simulink model "EA2_2_regulation_FIXED"  (R2024b)
settings: Solver=VariableStepAuto  StartTime=0.0  StopTime=T_SIM  RelTol=1e-3
values from neighbouring files (symbols this model uses):
  control_par = [k_1, k_2, k_3]    [EA2_2_regulation_FIXED.m]
  controller_index = 2    [EA2_2_regulation_FIXED.m]
  d = d_nominal    (= 0.165)    [EA2_2_regulation_FIXED.m]
  D = diag([0.001, 0.001, 0.0175/6, 0.0175/6, 0.0175/6, 0.0175/6*Ts, 0.0175/6*Ts].^2)    [EA2_2_regulation_FIXED.m]
  d_actual = d_nominal    (= 0.165)    [EA2_2_regulation_FIXED.m]
  ekf_online = 1    [EA2_2_regulation_FIXED.m]
  omega_M = 12    [EA2_2_regulation_FIXED.m]
  P_INIT_EKF = diag([0.001, 0.001, 0.0175/6, 0.0175/6, 0.0175/6, 0.0175/6*Ts, 0.0175/6*Ts].^2)    [EA2_2_regulation_FIXED.m]
  prob_gps_loss = 0    [EA2_2_regulation_FIXED.m]
  q_d = [2;2;0]    [EA2_2_regulation_FIXED.m]
  Q_INIT = [0;0;0]    [EA2_2_regulation_FIXED.m]
  r = r_nominal    (= 0.03)    [EA2_2_regulation_FIXED.m]
  R_2 = diag([ENCODER_QUANTIZATION/6,ENCODER_QUANTIZATION/6].^2)    [EA2_2_regulation_FIXED.m]
  R_5 = diag(([0.001, 0.001, 0.001, ENCODER_QUANTIZATION/6,ENCODER_QUANTIZATION/6]).^2)    [EA2_2_regulation_FIXED.m]
  r_actual = r_nominal    (= 0.03)    [EA2_2_regulation_FIXED.m]
  Ts = 0.04    [EA2_2_regulation_FIXED.m]
  Z_INIT_EKF = [Q_INIT; 0; 0; 0; 0]    [EA2_2_regulation_FIXED.m]
undefined symbols (not defined in the file or in its folder): w_max, X, Y
libraries: robotlib x4
settings Model: Creator=riccardo01  LastModifiedBy=Enrico
settings DataIOCC: SaveFormat=Array  ReturnWorkspaceOutputs=off
settings DebuggingCC: AlgebraicLoopMsg=none

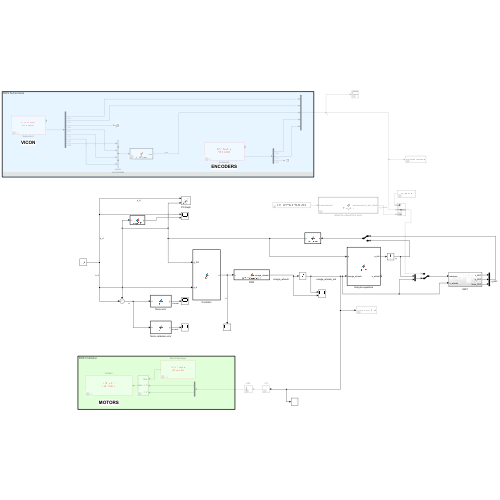
[thumbnail: Simulink's stored preview of the top-level diagram]
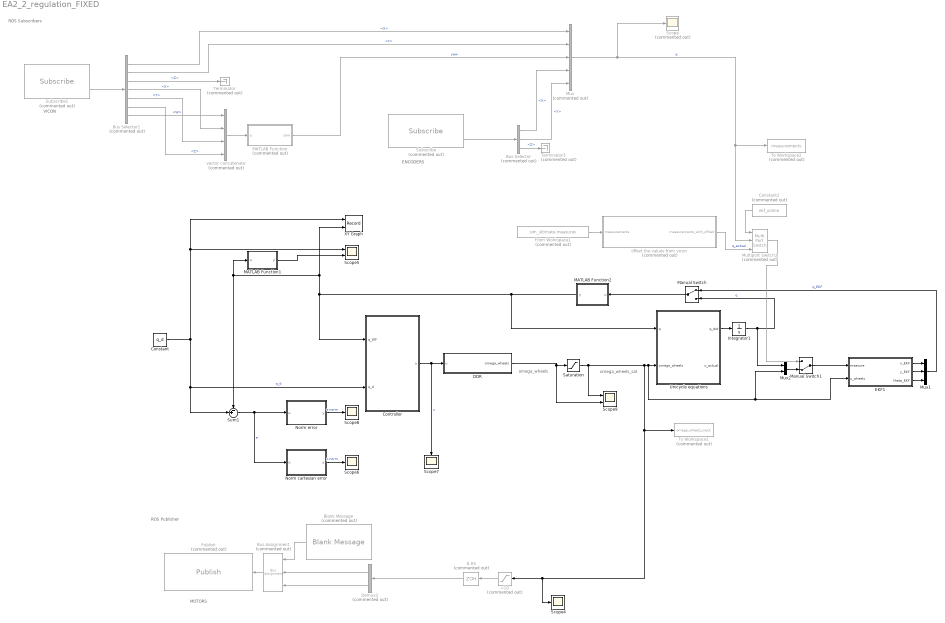
== system EA2_2_regulation_FIXED ==
  note: MOTORS
  note: ROS Publisher
  note: ENCODERS
  note: VICON
  note: ROS Subscribers
  note: omega_wheels
  note: omega_wheels_sat
  0.04 : ZeroOrderHold  Commented=on  SampleTime=Ts
  <10 : Saturate  Commented=on  UpperLimit=w_max  LowerLimit=-w_max
  Blank Message : robotlib/Blank Message  Commented=on  messageClass=Message  entityType=geometry_msgs/Vector3  messageType=geometry_msgs/Vector3  SampleTime=Ts  legacyBusStruct=off
      settings: LibrarySourceBlock=roslib/ROS/Blank Message
  Bus Assignment : BusAssignment  Commented=on  AssignedSignals=X,Y
  Bus Selector : BusSelector  Commented=on  OutputSignals=X,Y,Z
  Bus Selector1 : BusSelector  Commented=on  OutputSignals=Pose.Pose.Position.X,Pose.Pose.Position.Y,Pose.Pose.Position.Z,Pose.Pose.Orientation.X,Pose.Pose.Orientation.Y,Pose.Pose.Orientation.Z,Pose.Pose.Orientation.W
  Constant : Constant  Value=q_d
  Constant2 : Constant  Commented=on  Value=ekf_online
  Controller : MATLAB Function  TreatAsAtomicUnit=on
  DDR : MATLAB Function  TreatAsAtomicUnit=on
  Demux2 : Demux  Commented=on  Outputs=2
  EKF1 : Subsystem
  From Workspace1 : FromWorkspace  Commented=on  VariableName=sim_ultimate.measures
  Integrator1 : Integrator  InitialCondition=Q_INIT
  MATLAB Function : MATLAB Function  Commented=on  TreatAsAtomicUnit=on
  MATLAB Function1 : MATLAB Function  TreatAsAtomicUnit=on
  MATLAB Function2 : MATLAB Function  TreatAsAtomicUnit=on
  Manual Switch : ManualSwitch
  Manual Switch1 : ManualSwitch  CurrentSetting=0
  Multiport Switch2 : MultiPortSwitch  Commented=on  Inputs=2  SaturateOnIntegerOverflow=off  InputSameDT=off
  Mux : Mux  Commented=on  Inputs=5
  Mux1 : Mux  Inputs=3
  Mux2 : Mux  Inputs=2
  Norm cartesian error : MATLAB Function  TreatAsAtomicUnit=on
  Norm error : MATLAB Function  TreatAsAtomicUnit=on
  Publish : robotlib/Publish  Commented=on  topicSource=Specify your own  topic=/turtlebot_07/cmd_wheels  messageType=geometry_msgs/Vector3  legacyBusStruct=off  messageQueueLength=1
      settings: LibrarySourceBlock=roslib/ROS/Publish
  Saturation : Saturate  UpperLimit=omega_M  LowerLimit=-omega_M
  Scope : Scope  Commented=on
  Scope{4,6..8} (4 alike) : Scope
  Scope5 : Scope  NumInputPorts=2
  Scope9 : Scope  NumInputPorts=2
  Subscribe : robotlib/Subscribe  Commented=on  topicSource=Specify your own  topic=/turtlebot_07/wheelSpeeds  messageType=geometry_msgs/Vector3  SampleTime=-1  legacyBusStruct=off  messageQueueLength=1
      settings: LibrarySourceBlock=roslib/ROS/Subscribe
  Subscribe1 : robotlib/Subscribe  Commented=on  topicSource=Specify your own  topic=/turtlebot_07/odom  messageType=nav_msgs/Odometry  SampleTime=-1  legacyBusStruct=off  messageQueueLength=1
      settings: LibrarySourceBlock=roslib/ROS/Subscribe
  Sum1 : Sum  Inputs=-+|
  Terminator : Terminator  Commented=on
  Terminator3 : Terminator  Commented=on
  To Workspace1 : ToWorkspace  Commented=on  VariableName=omega_wheels_input  SampleTime=-1
  To Workspace2 : ToWorkspace  Commented=on  VariableName=measurements  SampleTime=-1
  Unicycle equations : MATLAB Function  TreatAsAtomicUnit=on
  XY Graph : Record  FileSettingsInternal="{\"entries\":[{\"content\":{\"excelSettings\":{\"content\":{},\"type\":\"Streamout.ExcelSettings\"}},\"type\":\"Streamout.FileSettingStorage\",\"uuid\":\"\"}],\"packageUris\":[\"http:\\/\\/schema.mathworks.com\\/mf0\\/streamout_blocks\\/R2020a\"],\"version\":\"1.0\"}"  Layout=[1 2]  SignalsInternal="{\"entries\":[{\"content\":{\"signals\":[{\"content\":{\"blockPath\":[],\"dimensions\":[3,1],\"domain\":\"\",\"hasChildren\":true,\"lineColor\":\"#fe330a\",\"lineWidth\":2,\"port\":2,\"sid\":[\"\"],\"signalID\":1,\"signalName\":\"MATLAB Function2\"},\"type\":\"RecordBlkView.Signal\",\"uuid\":\"\"},{\"content\":{\"blockPath\":[],\"channel\":[1,1],\"dimensions\":[3,1],\"domain\":\"\",\"lineColor\":\"#000000\",\"lineStyle\":\"DASH_DOT\",\"parentID\":1,\"plots\":[ 1 ],\"port\":2,\"sid\":[\"\"],\"signalID\":2,\"signalName\":\"MATLAB Function2\"},\"type\":\"RecordBlkView.Signal\",\"uuid\":\"\"},{\"content\":{\"blockPath\":[],\"dimensions\":[1,1],\"domain\":\"\",\"lineColor\":\"#77ac30\",\"lineWidth\":2,\"port\":1,\"sid\":[\"\"],\"signalID\":3,\"signalName\":\"x_EKF\"},\"type\":\"RecordBlkView.Signal\",\"uuid\":\"\"},{\"content\":{\"blockPath\":[],\"dimensions\":[1,1],\"domain\":\"\",\"lineColor\":\"#4dbeee\",\"lineWidth\":2,\"port\":2,\"sid\":[\"\"],\"signalID\":4,\"signalName\":\"y_EKF\"},\"type\":\"RecordBlkView.Signal\",\"uuid\":\"\"},{\"content\":{\"blockPath\":[],\"dimensions\":[3],\"domain\":\"\",\"hasChildren\":true,\"lineColor\":\"#edb120\",\"lineWidth\":2,\"port\":1,\"sid\":[\"\"],\"signalID\":5,\"signalName\":\"q_d\"},\"type\":\"RecordBlkView.Signal\",\"uuid\":\"\"},{\"content\":{\"blockPath\":[],\"channel\":[1],\"dimensions\":[3],\"domain\":\"\",\"lineColor\":\"#d95319\",\"parentID\":5,\"plots\":[ 1 ],\"port\":1,\"sid\":[\"\"],\"signalID\":6,\"signalName\":\"q_d\"},\"type\":\"RecordBlkView.Signal\",\"uuid\":\"\"},{\"content\":{\"blockPath\":[],\"channel\":[2,1],\"dimensions\":[3,1],\"domain\":\"\",\"lineColor\":\"#edb120\",\"lineWidth\":2,\"parentID\":1,\"plots\":[ 1 ],\"port\":2,\"sid\":[\"\"],\"signalID\":7,\"signalName\":\"MATLAB Function2\"},\"type\":\"RecordBlkView.Signal\",\"uuid\":\"\"},{\"content\":{\"blockPath\":[],\"channel\":[3,1],\"dimensions\":[3,1],\"domain\":\"\",\"lineColor\":\"#7e2f8e\",\"lineWidth\":2,\"parentID\":1,\"plots\":[ 2, 9 ],\"port\":2,\"sid\":[\"\"],\"signalID\":8,\"signalName\":\"MATLAB Function2\"},\"type\":\"RecordBlkView.Signal\",\"uuid\":\"\"},{\"content\":{\"blockPath\":[],\"channel\":[2],\"dimensions\":[3],\"domain\":\"\",\"lineColor\":\"#77ac30\",\"parentID\":5,\"plots\":[ 1 ],\"port\":1,\"sid\":[\"\"],\"signalID\":9,\"signalName\":\"q_d\"},\"type\":\"RecordBlkView.Signal\",\"uuid\":\"\"},{\"content\":{\"blockPath\":[],\"channel\":[3],\"dimensions\":[3],\"domain\":\"\",\"lineColor\":\"#4dbeee\",\"parentID\":5,\"plots\":[ 2, 9 ],\"port\":1,\"sid\":[\"\"],\"signalID\":10,\"signalName\":\"q_d\"},\"type\":\"RecordBlkView.Signal\",\"uuid\":\"\"}]},\"type\":\"RecordBlkView.InputSignals\",\"uuid\":\"\"}],\"packageUris\":[\"http:\\/\\/schema.mathworks.com\\/mf0\\/streamout_blocks\\/R2020a\"],\"version\":\"1.0\"}"  VisualizationBindings="{\"xyplotplugin\":{\"info\":[{\"series\":[{\"bindingParametersList\":[{\"parameter\":\"X-Axis\",\"signalID\":6,\"signalName\":\"q_d(1)\"},{\"parameter\":\"Y-Axis\",\"signalID\":9,\"signalName\":\"q_d(2)\"}],\"seriesID\":0},{\"bindingParametersList\":[{\"parameter\":\"X-Axis\",\"signalID\":2,\"signalName\":\"MATLAB Function2(1,1)\"},{\"parameter\":\"Y-Axis\",\"signalID\":7,\"signalName\":\"MATLAB Function2(2,1)\"}],\"seriesID\":1}],\"subplotID\":1}]}}"  CompatibilityTag=XY
  offset the values from vicon : MATLAB Function  Commented=on  TreatAsAtomicUnit=on
  vector concatenate : Concatenate  Commented=on  NumInputs=4
  wires:
  0.04/1 -> Demux2/1
  Blank Message/1 -> Bus Assignment/1
  <10/1 -> 0.04/1
  Demux2/2 -> Bus Assignment/3
  Bus Assignment/1 -> Publish/1
  Demux2/1 -> Bus Assignment/2
  vector concatenate/1 -> MATLAB Function/1(q)
  Subscribe/2 -> Bus Selector/1
  Bus Selector1/5 -> vector concatenate/3  "<Y>"
  Bus Selector/2 -> Mux/5  "<Y>"
  Bus Selector1/3 -> Terminator/1  "<Z>"
  Bus Selector1/1 -> Mux/1  "<X>"
  MATLAB Function/1(yaw) -> Mux/3  "yaw"
  Subscribe1/2 -> Bus Selector1/1
  Bus Selector1/6 -> vector concatenate/4  "<Z>"
  Bus Selector/1 -> Mux/4  "<X>"
  Mux/1 -> Scope/1, To Workspace2/1, Multiport Switch2/2  "q"
  Bus Selector/3 -> Terminator3/1  "<Z>"
  Bus Selector1/2 -> Mux/2  "<Y>"
  Bus Selector1/7 -> vector concatenate/1  "<W>"
  Bus Selector1/4 -> vector concatenate/2  "<X>"
  From Workspace1/1 -> offset the values from vicon/1(measurements)
  offset the values from vicon/1(measurements_with_offset) -> Multiport Switch2/3  "q_actual"
  Constant2/1 -> Multiport Switch2/1
  Norm error/1(y) -> Scope8/1  "e norm"
  Norm cartesian error/1(y) -> Scope6/1  "p norm"
  Controller/1(u) -> Scope7/1, DDR/1(u)  "u"
  Unicycle equations/1(q_dot) -> Integrator1/1
  MATLAB Function1/1(y) -> Scope5/2
  Sum1/1 -> Norm cartesian error/1(u), Norm error/1(u)  "e"
  DDR/1(omega_wheels) -> Saturation/1, Scope9/2
  MATLAB Function2/1(y) -> Unicycle equations/1(q), Sum1/1, MATLAB Function1/1(u), XY Graph/2, Controller/1(q_WF)
  Saturation/1 -> Scope4/1, <10/1, To Workspace1/1, EKF1/2(u_wheels), Mux2/2, Unicycle equations/2(omega_wheels), Scope9/1
  Constant/1 -> Sum1/2, Controller/2(q_d), XY Graph/1, Scope5/1  "q_d"
  EKF1/1(x_EKF) -> Mux1/1
  EKF1/2(y_EKF) -> Mux1/2
  EKF1/3(theta_EKF) -> Mux1/3
  Integrator1/1 -> Mux2/1, Manual Switch/2  "q"
  Mux1/1 -> Manual Switch/1  "q_EKF"
  Manual Switch/1 -> MATLAB Function2/1(u)
  Multiport Switch2/1 -> Manual Switch1/1
  Manual Switch1/1 -> EKF1/1(measure)
  Mux2/1 -> Manual Switch1/2

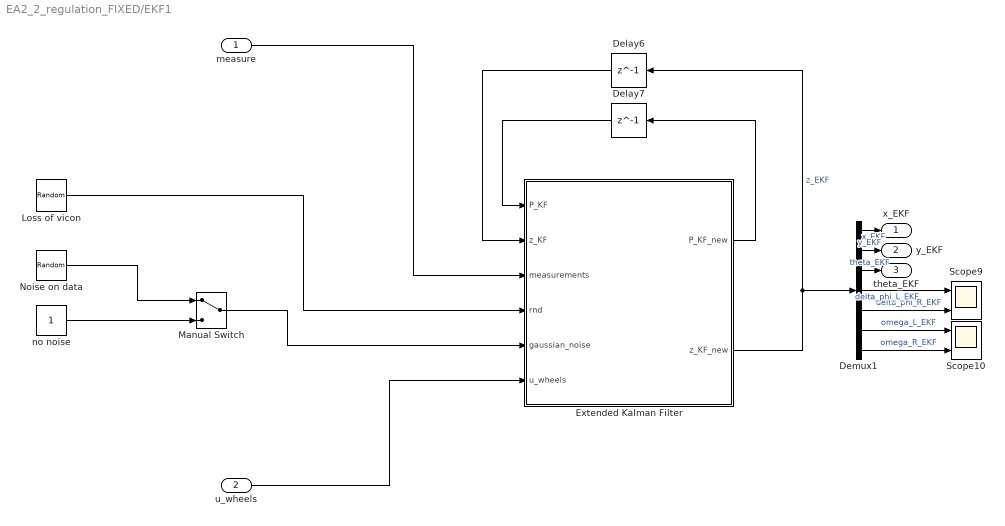
== system EA2_2_regulation_FIXED/EKF1 ==
  measure : Inport
  u_wheels : Inport  Port=2
  " Loss of vicon" : UniformRandomNumber  Minimum=0
  Delay6 : Delay  DelayLength=1  InitialCondition=Z_INIT_EKF
  Delay7 : Delay  DelayLength=1  InitialCondition=P_INIT_EKF
  Demux1 : Demux  Outputs=7
  Extended Kalman Filter : MATLAB Function  TreatAsAtomicUnit=on
  Manual Switch : ManualSwitch
  Noise on data : RandomNumber  Variance=0.0001
  Scope10 : Scope  NumInputPorts=2
  Scope9 : Scope  NumInputPorts=2
  no noise : Constant
  x_EKF : Outport
  y_EKF : Outport  Port=2
  theta_EKF : Outport  Port=3
  wires:
  Demux1/6 -> Scope10/1  "omega_L_EKF"
  Demux1/3 -> theta_EKF/1  "theta_EKF"
  Delay6/1 -> Extended Kalman Filter/2(z_KF)
  Delay7/1 -> Extended Kalman Filter/1(P_KF)
  Noise on data/1 -> Manual Switch/1
  Demux1/5 -> Scope9/2  "delta_phi_R_EKF"
  Demux1/7 -> Scope10/2  "omega_R_EKF"
  Extended Kalman Filter/1(P_KF_new) -> Delay7/1
  Manual Switch/1 -> Extended Kalman Filter/5(gaussian_noise)
  " Loss of vicon"/1 -> Extended Kalman Filter/4(rnd)
  Demux1/1 -> x_EKF/1  "x_EKF"
  Demux1/4 -> Scope9/1  "delta_phi_L_EKF"
  no noise/1 -> Manual Switch/2
  u_wheels/1 -> Extended Kalman Filter/6(u_wheels)
  Extended Kalman Filter/2(z_KF_new) -> Demux1/1, Delay6/1  "z_EKF"
  measure/1 -> Extended Kalman Filter/3(measurements)
  Demux1/2 -> y_EKF/1  "y_EKF"

== matlab function EA2_2_regulation_FIXED/Norm error ==
  data: u input; y output
function y = fcn(u)
y = [u(1);u(2); wrapToPi(u(3))];

== matlab function EA2_2_regulation_FIXED/Unicycle equations ==
  data: q input; omega_wheels input; q_dot output; r_actual parameter; d_actual parameter; u_actual output
function [q_dot, u_actual] = q_dot(q, omega_wheels, r_actual, d_actual)
u_actual = [r_actual/2, r_actual/2;-r_actual/d_actual, r_actual/d_actual]*omega_wheels;
theta = q(3);
q_dot = [[cos(theta), 0];[sin(theta), 0];[0,1]]*u_actual;

== matlab function EA2_2_regulation_FIXED/Controller ==
  data: q_WF input; q_d input; u output; controller_index parameter; control_par parameter
function u = fcn(q_WF, q_d, controller_index, control_par)

% roto translation
omega_d = q_d(3);
e = q_WF - q_d;
q_WF(1) = cos(omega_d)*e(1) + sin(omega_d)*e(2);
q_WF(2) = -sin(omega_d)*e(1) + cos(omega_d)*e(2);
q_WF(3) = e(3);


% select the controller
if controller_index == 1
    % cartesian regulator
    % transform q_WF
    % compute the input
    e_p = [-q_WF(1); -q_WF(2)];
    n = [cos(q_WF(3)); sin(q_WF(3))];
    % pointing error
    gamma = wrapToPi(atan2(q_WF(2),q_WF(1)) + pi - q_WF(3));

    v = control_par(1) * (e_p' * n);
    omega = control_par(2) * gamma;
    u = [v;omega];

else
    % posture regulator
    % transform q_WF
    % compute pointing error

    ro = sqrt(q_WF(1)^2 + q_WF(2)^2);
    % pointing error
    gamma = wrapToPi(atan2(q_WF(2),q_WF(1)) + pi - q_WF(3));
    delta = wrapToPi(gamma + q_WF(3));
    
    v = control_par(1) * ro * cos(gamma);

    if abs(gamma)<1e-4
        omega = control_par(2)*gamma + control_par(1)*cos(gamma)*(gamma + control_par(3)*delta);
    else
        omega = control_par(2)*gamma + control_par(1)*sin(gamma)*cos(gamma)*(gamma + control_par(3)*delta)/gamma;
    end
    
    u = [v;omega];
end

== matlab function EA2_2_regulation_FIXED/DDR ==
  data: u input; omega_wheels output; r parameter; d parameter; omega_M parameter
function omega_wheels = kin2omegawheels(u, r, d, omega_M)
omega_l = u(1)/r-d/(2*r)*u(2);
omega_r = u(1)/r+d/(2*r)*u(2);

if (abs(omega_l) > omega_M) || (abs(omega_r) > omega_M)
    omega_prop = max(abs(omega_l), abs(omega_r));
    omega_l = omega_l*omega_M/omega_prop;
    omega_r = omega_r*omega_M/omega_prop;
end
omega_wheels = [omega_l;omega_r];

== matlab function EA2_2_regulation_FIXED/offset the values from vicon ==
  data: measurements input; measurements_with_offset output; Q_INIT parameter
function measurements_with_offset  = offset_vicon(measurements, Q_INIT)

persistent initial_vicon_pose;
persistent first_run;

% Record first vicon measurement as reference and use it for offset
if isempty(first_run)
    first_run = false;
    initial_vicon_pose = [measurements(1); measurements(2); measurements(3)];
end

% relative transformation from initial vicon pose
delta_x     = measurements(1) - initial_vicon_pose(1);
delta_y     = measurements(2) - initial_vicon_pose(2);
delta_angle = measurements(3) - initial_vicon_pose(3);


% rotation matrix to account for angle offset
rot_matrix = [cos(Q_INIT(3)), -sin(Q_INIT(3));
              sin(Q_INIT(3)),  cos(Q_INIT(3))];

% transform position
rotated_xy = rot_matrix * [delta_x; delta_y];

% fliping the theta because it shows wrong
delta_angle = -delta_angle;
rotated_xy(1) = -rotated_xy(1);

measurements_with_offset = measurements;
measurements_with_offset(1) = Q_INIT(1) + rotated_xy(1);
measurements_with_offset(2) = Q_INIT(2) + rotated_xy(2);
measurements_with_offset(3) = Q_INIT(3) + delta_angle;
end

== matlab function EA2_2_regulation_FIXED/EKF1/Extended Kalman Filter ==
  data: P_KF input; P_KF_new output; z_KF input; measurements input; D parameter; R_2 parameter; R_5 parameter; Ts parameter; r parameter; d parameter; prob_gps_loss parameter; rnd input; gaussian_noise input; z_KF_new output; u_wheels input
function [P_KF_new, z_KF_new] = EKF_filtering(P_KF, z_KF, measurements, D, R_2, R_5 ,Ts, r, d, prob_gps_loss, rnd, gaussian_noise,u_wheels)


% z_KF = [x_EKF, y_EKF, theta_EKF, delta_phi_L_EKF, delta_phi_R_EKF, omega_L_EKF, omega_R_EKF]

v_k = r * (z_KF(6) + z_KF(7))/2;
w_k = r * (z_KF(7) - z_KF(6))/d;

theta_mean = z_KF(3) + (w_k * Ts)/2;

F_k = [1, 0, -Ts * v_k * sin(theta_mean), 0, 0, Ts * r * cos(theta_mean)/2 + (Ts)^2 * r * v_k * sin(theta_mean)/(2*d), Ts * r * cos(theta_mean)/2 - (Ts)^2 * r * v_k * sin(theta_mean)/(2*d);
       0, 1,  Ts * v_k * cos(theta_mean), 0, 0, Ts * r * sin(theta_mean)/2 + (Ts)^2 * r * v_k * cos(theta_mean)/(2*d), Ts * r * sin(theta_mean)/2 - (Ts)^2 * r * v_k * cos(theta_mean)/(2*d);
       0, 0, 1, 0, 0, (-Ts*r)/d, (Ts*r)/d;
       0, 0, 0, 0, 0, Ts, 0;
       0, 0, 0, 0, 0, 0, Ts;
       0, 0, 0, 0, 0, 0, 0;
       0, 0, 0, 0, 0, 0, 0];

%% Prediction part

z_pred = [z_KF(1)+(Ts*r*(z_KF(6)+z_KF(7))/2)*cos(theta_mean + (Ts*r*(z_KF(6)+z_KF(7)))/(2*d));
          z_KF(2)+(Ts*r*(z_KF(6)+z_KF(7))/2)*sin(theta_mean + (Ts*r*(z_KF(7)-z_KF(6)))/(2*d));
          theta_mean + (Ts*r*(z_KF(7)-z_KF(6))/(2*d));
          Ts*z_KF(6);
          Ts*z_KF(7);
          u_wheels(1);
          u_wheels(2)];

P_pred = F_k * P_KF * F_k' + D;


%% Update

if(rnd<prob_gps_loss)

    % Just encoders
    y_measurement = [measurements(4); measurements(5)];
    H = [0, 0, 0, 0, 0, 1, 0;
         0, 0, 0, 0, 0, 0, 1];

    e = y_measurement - H * z_pred;
    K = P_pred * H' /(H * P_pred * H' + R_2);

    z_KF_new = z_pred +  K * e;
    P_KF_new = P_pred - K * H * P_pred;

else 
    % GPS(x,y,yaw) + Encoders(omegaL,omegaR)
    y_measurement = [measurements(1)+gaussian_noise;measurements(2)+gaussian_noise;measurements(3)+gaussian_noise; measurements(4); measurements(5)];
    
    H = [1, 0, 0, 0, 0, 0, 0;
         0, 1, 0, 0, 0, 0, 0;
         0, 0, 1, 0, 0, 0, 0;
         0, 0, 0, 0, 0, 1, 0;
         0, 0, 0, 0, 0, 0, 1];

    e = y_measurement - H * z_pred;
    K = P_pred * H' /(H * P_pred * H' + R_5);

    z_KF_new = z_pred + K * e;
    P_KF_new = P_pred - K * H * P_pred;
end

end

== matlab function EA2_2_regulation_FIXED/MATLAB Function ==
  data: q input; yaw output
function yaw = quat2yaw(q)

% normalize to avoid issues
q = q / norm(q);

w = q(1);
x = q(2);
y = q(3);
z = q(4);

% rotation around Z axis
yaw = atan2(2*(w*z + x*y), 1 - 2*(y^2 + z^2));

end

== matlab function EA2_2_regulation_FIXED/MATLAB Function1 ==
  data: u input; y output
function y  = wrapToPi(u)
%theta = wrapToPi(u(3));
%theta = unwrap(u(3));
theta = u(3);
y = [u(1),u(2),theta]';

== matlab function EA2_2_regulation_FIXED/MATLAB Function2 ==
  data: u input; y output
function y  = wrapToPi(u)
%theta = wrapToPi(u(3));
%theta = unwrap(u(3));
theta = u(3);
y = [u(1),u(2),theta]';

== matlab function EA2_2_regulation_FIXED/Norm cartesian error ==
  data: u input; y output
function y = fcn(u)

y = sqrt(sum(u(1:2).^2));
